simulink subsystem "CqdotqMatrix"  (R2024b)
settings: Solver=VariableStepAuto  StartTime=0.0  StopTime=10.0  RelTol=1e-3
undefined symbols (not defined in the file or in its folder): body, mot, wheel
settings Model: Creator=federico  LastModifiedBy=federico

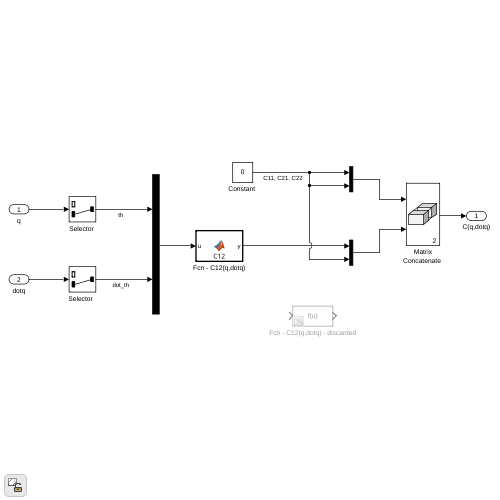
[thumbnail: Simulink's stored preview of the top-level diagram]
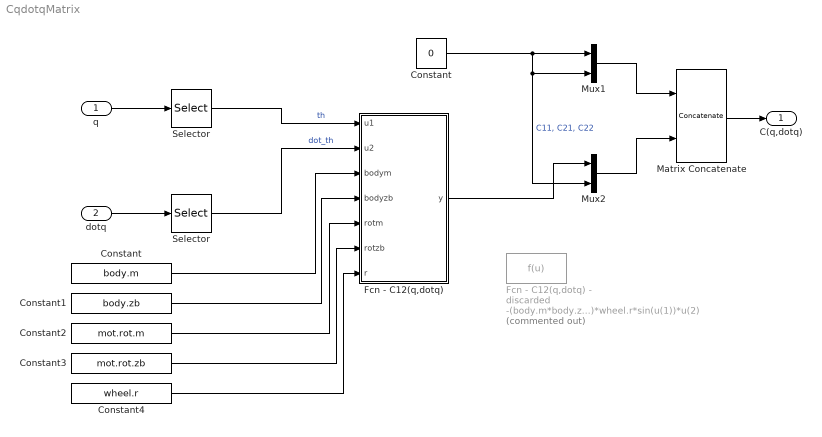
== system CqdotqMatrix ==
  q : Inport
  dotq : Inport  Port=2
  Constant : Constant  Value=body.m
  "Constant " : Constant  Value=0
  Constant1 : Constant  Value=body.zb
  Constant2 : Constant  Value=mot.rot.m
  Constant3 : Constant  Value=mot.rot.zb
  Constant4 : Constant  Value=wheel.r
  Fcn - C12(q,dotq) : MATLAB Function  TreatAsAtomicUnit=on
  Fcn - C12(q,dotq) - discarded : Fcn  Commented=on  Expr=-(body.m*body.zb + 2*mot.rot.m*mot.rot.zb)*wheel.r*sin(u(1))*u(2)
  "Matrix Concatenate " : Concatenate  Mode=Multidimensional array  ConcatenateDimension=2
  Mux1 : Mux  Inputs=2
  Mux2 : Mux  Inputs=2
  "Selector " : Selector  InputPortWidth=2  IndexOptions=Index vector (dialog)  Indices=[2]  OutputSizes=1
  "Selector  " : Selector  InputPortWidth=2  IndexOptions=Index vector (dialog)  Indices=[2]  OutputSizes=1
  C(q,dotq) : Outport
  wires:
  q/1 -> "Selector "/1
  dotq/1 -> "Selector  "/1
  "Selector "/1 -> Fcn - C12(q,dotq)/1(u1)  "th"
  "Selector  "/1 -> Fcn - C12(q,dotq)/2(u2)  "dot_th"
  Fcn - C12(q,dotq)/1(y) -> Mux2/1
  "Constant "/1 -> Mux2/2, Mux1/2, Mux1/1  "C11, C21, C22"
  Mux1/1 -> "Matrix Concatenate "/1
  Mux2/1 -> "Matrix Concatenate "/2
  "Matrix Concatenate "/1 -> C(q,dotq)/1
  Constant/1 -> Fcn - C12(q,dotq)/3(bodym)
  Constant1/1 -> Fcn - C12(q,dotq)/4(bodyzb)
  Constant2/1 -> Fcn - C12(q,dotq)/5(rotm)
  Constant3/1 -> Fcn - C12(q,dotq)/6(rotzb)
  Constant4/1 -> Fcn - C12(q,dotq)/7(r)

== matlab function CqdotqMatrix/Fcn - C12(q,dotq) ==
  data: u1 input; y output; u2 input; bodym input; bodyzb input; rotm input; rotzb input; r input
function y = C12(u1,u2,bodym, bodyzb, rotm, rotzb, r)

y = -(bodym*bodyzb + 2*rotm*rotzb)*r*sin(u1)*u2;
